simulink model "Q1_1"  (R2020b)
settings: Solver=VariableStepAuto  StartTime=0.0  StopTime=10.0  RelTol=1e-3
settings Model: Creator=DELL  LastModifiedBy=DELL

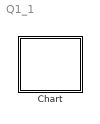
== system Q1_1 ==
  Chart : Stateflow chart  TreatAsAtomicUnit=on

== stateflow chart Q1_1/Chart ==
  state Qa0
    (default) -> (junction 10) : % When Qa=0
    (junction 10) -> (junction 11) [order 1] : [Qc==0]
    (junction 11) -> (junction 13) : {Qa_new=0,Qb_new=Qb,Qc_new=1;}
    (junction 10) -> (junction 15) [order 2]
    (junction 15) -> (junction 12) [order 2] : [Qb==1]{Qa_new=0,Qb_new=0,Qc=0;}
    (junction 15) -> (junction 12) [order 1] : [Qb==0]{Qa_new=0,Qb_new=1,Qc=0;}
    (junction 13) -> (junction 12)
    (junction 12) -> (junction 14)
  state Qa1
    entry:
    Qa_new=Qa;
    Qb_new=Qb;
    Qc_new=Qc;
  (default) -> Qa0
  Qa0 -> Qa1 : [Qa==1]
